simulink model "MT_FOC_control_autotuning"  (R2018a)
settings: Solver=ode4  StartTime=0.0  StopTime=3  FixedStep=1e-6  MaxStep=1e-4  RelTol=1e-3
undefined symbols (not defined in the file or in its folder): sigbuilder_block
libraries: powerlib x10, peTransforms x2, powerlib_meascontrol x1
settings Model: Creator=Admin  LastModifiedBy=Admin
settings DebuggingCC: MaxConsecutiveZCsMsg=none

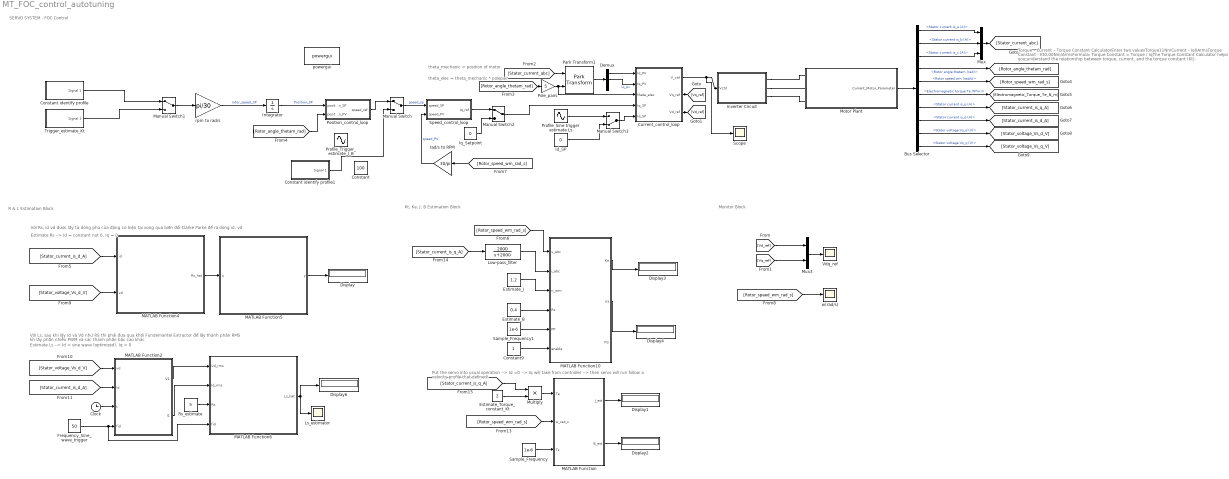
== system MT_FOC_control_autotuning ==
  note: Monitor Block
  note: Put the servo into usual operation --> Id =0 --> Iq will take from controller --> then servo will run follow a velocity profile that defined!
  note: Kt, Ke, J, B Estimation Block
  note: R & L Estimation Block
  note: Estimate Rs --> Id = constant not 0, Iq = 0
  note: SERVO SYSTEM - FOC Control
  note: Với Ls, sau khi lấy Id và Vd như RS thì phải đưa qua khối Fundemantel Extractor để lấy thành phần RMS kh lấy phần nhiễu PWM và các thành phần bậc cao khác
  note: Với Rs, id vd được lấy từ dòng pha của động cơ hiện tại xong qua biến đổi Clarke Parke để ra dòng id, vd
  note: Torque – Current – Torque Constant CalculatorEnter two valuesTorque11NmCurrent - Iq0ArmsTorque Constant - Kt0.00Nm/ArmsFormula: Torque Constant = Torque / IqThe Torque Constant Calculator helps you understand the relationship between torque, current, and the torque constant (Kt​).
  note: theta_mechanic = position of motor
  note: theta_elec = theta_mechanic * polepair
  note: Estimate Ls --> Id = sine wave (optimized), Iq = 0
  Bus Selector : BusSelector  OutputSignals=Stator current is_a (A),Stator current is_b (A),Stator current is_c (A),Rotor angle thetam (rad),Rotor speed wm (rad/s),Electromagnetic torque Te (N*m),Stator current is_q (A),Stator current is_d (A),Stator voltage Vs_d (V),Stator voltage Vs_q (V)
  Clock : Clock
  Constant : Constant  Value=100
  Constant identify profile : Subsystem  Tag=STV Subsys  LoadFcn=sigbuilder_block('load');  StartFcn=sigbuilder_block('start');  StopFcn=sigbuilder_block('stop');  ClipboardFcn=sigbuilder_block('clipboard');  mask(Sigbuilder block){tuvar=[0:10]}
      mask help: Simulink:masks:SigbuilderBlock_MD
      mask init:
      | if ~strcmp(get_param(bdroot(gcbh),'SimulationStatus'),'stopped') tuvar = sigbuilder_block('maskInit'); end
      settings: CopyFcn=sigbuilder_block('copy');  DeleteFcn=sigbuilder_block('delete');  ModelCloseFcn=sigbuilder_block('modelClose');  PreSaveFcn=sigbuilder_block('preSave');  PauseFcn=sigbuilder_block('pause');  ContinueFcn=sigbuilder_block('continue');  NameChangeFcn=sigbuilder_block('namechange');  OpenFcn=sigbuilder_block('open',[356.4 94.8 550.8 400.2 ]);  CloseFcn=sigbuilder_block('close');
      mask Display: plot(0, 0, 100, 100,[2, 2, 32, 32, 2], [68, 8, 8, 68, 68],[32, 2], [38, 38], [32, 19, 2],[53, 60, 44], [32, 17, 17, 2],[16, 16, 31, 31]);txt = getActiveGroup(gcbh);text(2, 100, txt,'verticalAlignment', 'top');
  Constant identify profile1 : Subsystem  Tag=STV Subsys  LoadFcn=sigbuilder_block('load');  StartFcn=sigbuilder_block('start');  StopFcn=sigbuilder_block('stop');  ClipboardFcn=sigbuilder_block('clipboard');  mask(Sigbuilder block){tuvar=[0:10]}
      mask help: Simulink:masks:SigbuilderBlock_MD
      mask init:
      | if ~strcmp(get_param(bdroot(gcbh),'SimulationStatus'),'stopped') tuvar = sigbuilder_block('maskInit'); end
      settings: CopyFcn=sigbuilder_block('copy');  DeleteFcn=sigbuilder_block('delete');  ModelCloseFcn=sigbuilder_block('modelClose');  PreSaveFcn=sigbuilder_block('preSave');  PauseFcn=sigbuilder_block('pause');  ContinueFcn=sigbuilder_block('continue');  NameChangeFcn=sigbuilder_block('namechange');  OpenFcn=sigbuilder_block('open',[356.4 94.8 550.8 400.2 ]);  CloseFcn=sigbuilder_block('close');
      mask Display: plot(0, 0, 100, 100,[2, 2, 32, 32, 2], [68, 8, 8, 68, 68],[32, 2], [38, 38], [32, 19, 2],[53, 60, 44], [32, 17, 17, 2],[16, 16, 31, 31]);txt = getActiveGroup(gcbh);text(2, 100, txt,'verticalAlignment', 'top');
  Constant9 : Constant
  Current_control_loop : Subsystem  mask{Kp=100, Ki=10}
  Demux : Demux  Outputs=3
  Display{,1..4,6} (6 alike) : Display
  Estimate_B : Constant  Value=0.4
  Estimate_J : Constant  Value=1.2
  "Estimate_Torque_constant_Kt " : Constant  Value=2  VectorParams1D=off  SampleTime=-1
  Frequency_Sine_wave_trigger : Constant  Value=50
  Id_SP : Constant  Value=0
  Integrator : Integrator
  Inverter Circuit : Subsystem  mask{Vdc=300, f_triangle=10000}
      mask prompts: Vdc "DC supply"; f_triangle "Freq carry signal"
  Iq_Setpoint : Constant  Value=0
  Low-pass_filter : TransferFcn  Numerator=[2000]  Denominator=[1 2000]
  Ls_estimator : Scope
  MATLAB Function : MATLAB Function  TreatAsAtomicUnit=on
  MATLAB Function10 : MATLAB Function  TreatAsAtomicUnit=on
  MATLAB Function2 : MATLAB Function  TreatAsAtomicUnit=on
  MATLAB Function4 : MATLAB Function  TreatAsAtomicUnit=on
  MATLAB Function5 : MATLAB Function  TreatAsAtomicUnit=on
  MATLAB Function6 : MATLAB Function  TreatAsAtomicUnit=on
  Manual Switch : ManualSwitch
  Manual Switch1 : ManualSwitch
  Manual Switch2 : ManualSwitch
  Manual Switch3 : ManualSwitch  CurrentSetting=0
  Motor Plant : Subsystem  mask{Load=0, Stator_Rs=2.4, L=0.00334, Torque_constant=0.2, pole_pairs=5, Intertia=0.000034, B=0}
      mask prompts: Load "Input load to Motor? (N.m)"; Stator_Rs "Stator phase resistance Rs (ohm)?"; L "Stator Armature inductance (H)?"; Torque_constant "Torque_constant? (N.m/A_peak)"; pole_pairs "Pole_pairs? (np)"; Intertia "Intertia (kg.m^2)"; B "Statis friction constant (N.m.s)"
  Multiply : Product
  Mux : Mux  Inputs=3
  Mux3 : Mux  Inputs=2
  Park Transform1 : peTransforms/Park Transform  AxisAlignment=Q-axis  PowerInvariant=off
  Pole_pairs : Gain  Gain=5
  Position_control_loop : Subsystem  mask{Kp=100, Ki=10, Feed_Fw_gain=1}
  Profile_Sine trigger estimate Ls : Sin  Amplitude=3  Frequency=100*pi  SampleTime=0
  Profile_Trigger_estimate_J_B : Sin  Amplitude=100  SampleTime=0
  Rs_estimate : Constant  Value=5
  Sample_Frequency : Constant  Value=1e-6
  Sample_Frequency1 : Constant  Value=1e-6
  Scope : Scope
  Speed_control_loop : Subsystem  mask{Kp=100, Ki=10}
  Trigger_estimate_Kt : Subsystem  Tag=STV Subsys  LoadFcn=sigbuilder_block('load');  StartFcn=sigbuilder_block('start');  StopFcn=sigbuilder_block('stop');  ClipboardFcn=sigbuilder_block('clipboard');  mask(Sigbuilder block){tuvar=[0:10]}
      mask help: Simulink:masks:SigbuilderBlock_MD
      mask init:
      | if ~strcmp(get_param(bdroot(gcbh),'SimulationStatus'),'stopped') tuvar = sigbuilder_block('maskInit'); end
      settings: CopyFcn=sigbuilder_block('copy');  DeleteFcn=sigbuilder_block('delete');  ModelCloseFcn=sigbuilder_block('modelClose');  PreSaveFcn=sigbuilder_block('preSave');  PauseFcn=sigbuilder_block('pause');  ContinueFcn=sigbuilder_block('continue');  NameChangeFcn=sigbuilder_block('namechange');  OpenFcn=sigbuilder_block('open',[356.4 94.8 550.8 400.2 ]);  CloseFcn=sigbuilder_block('close');
      mask Display: plot(0, 0, 100, 100,[2, 2, 32, 32, 2], [68, 8, 8, 68, 68],[32, 2], [38, 38], [32, 19, 2],[53, 60, 44], [32, 17, 17, 2],[16, 16, 31, 31]);txt = getActiveGroup(gcbh);text(2, 100, txt,'verticalAlignment', 'top');
  Vdq_ref : Scope
  powergui : powerlib/powergui  Priority=1  SimulationMode=Discrete  SampleTime=1e-6  frequency=60  Iterations=50  frequencyindice=0  Pbase=100e6  ErrMax=1e-4  UnitsV=kV  UnitsW=MW  buscounter=0  FunctionMessages=off  echomessages=off  EnableUseOfTLC=off  CurrentSourceSwitches=off  DisableSnubberDevices=off  DisableRonSwitches=off  DisableVfSwitches=off  DisplayEquations=off  SolverType=Tustin/Backward Euler (TBE)  Interpol=off  ExternalGateDelay=off  methode=off  Ts=100  x0status=blocks  SPID=on  SwTol=0  HookPort=off  RestoreLinks=warning  ResistiveCurrentMeasurement=off  Frange=[0:2:500]  Ylog=off  Xlog=on  ShowGrid=off  save=off  variable=ZData  structure=0  ZoomFFT=off  StartTime=0.0  cycles=1  DisplayStyle=1  fundamental=60  FreqAxis=off  MaxFrequency=1000  frequencyindicesteady=1  RmsSteady=1  display=off
  rad/s to RPM : Gain  Gain=30/pi
  rpm to rad/s : Gain  Gain=pi/30
  w(rad/s) : Scope
  wires:
  Bus Selector/1 -> Mux/1  "<Stator current is_a (A)>"
  Bus Selector/2 -> Mux/2  "<Stator current is_b (A)>"
  Bus Selector/3 -> Mux/3  "<Stator current is_c (A)>"
  Pole_pairs/1 -> Current_control_loop/3("theta_elec "), Park Transform1/2
  Park Transform1/1 -> Demux/1
  rpm to rad/s/1 -> Integrator/1  "rotor_speed_SP"
  Integrator/1 -> Position_control_loop/1(position_SP)  "Position_SP"
  Position_control_loop/1(speed_ref) -> Manual Switch/1
  Bus Selector/6 -> [Electromagnetic_Torque_Te_N_m]  "<Electromagnetic torque Te (N*m)>"
  Sample_Frequency/1 -> MATLAB Function/3(Ts)
  Constant identify profile/1(Signal 1) -> Manual Switch1/1
  Manual Switch1/1 -> rpm to rad/s/1
  Speed_control_loop/1(Iq_ref) -> Manual Switch2/1
  Iq_Setpoint/1 -> Manual Switch2/2
  MATLAB Function4/1(Rs_hat) -> MATLAB Function5/1(u)
  Id_SP/1 -> Manual Switch3/2
  Profile_Sine trigger estimate Ls/1 -> Manual Switch3/1
  MATLAB Function6/1(Ls_hat) -> Display6/1, Ls_estimator/1
  Clock/1 -> MATLAB Function2/3(t)
  Low-pass_filter/1 -> MATLAB Function10/2(i_abc)
  Trigger_estimate_Kt/1(Signal 1) -> Manual Switch1/2
  Sample_Frequency1/1 -> MATLAB Function10/5(PP)
  Constant9/1 -> MATLAB Function10/6(enable)
  Motor Plant/1(Current_Motor_Parameter) -> Bus Selector/1
  [Vd_ref] -> Mux3/1
  Mux3/1 -> Vdq_ref/1
  [Vq_ref] -> Mux3/2
  Current_control_loop/1(V_ctrl) -> Scope/1, Inverter Circuit/1(Vctrl)
  Current_control_loop/2(Vq_ref) -> [Vq_ref]
  Current_control_loop/3(Vd_ref) -> [Vd_ref]
  [Stator_current_abc] -> Park Transform1/1
  Mux/1 -> [Stator_current_abc]
  Bus Selector/4 -> [Rotor_angle_thetam_rad]  "<Rotor angle thetam (rad)>"
  [Rotor_angle_thetam_rad] -> Pole_pairs/1
  [Rotor_angle_thetam_rad] -> Position_control_loop/2(position_PV)
  [Rotor_speed_wm_rad_s] -> MATLAB Function10/1(v_abc)
  [Rotor_speed_wm_rad_s] -> rad/s to RPM/1
  Bus Selector/5 -> [Rotor_speed_wm_rad_s]  "<Rotor speed wm (rad/s)>"
  [Rotor_speed_wm_rad_s] -> w(rad/s)/1
  Bus Selector/10 -> [Stator_voltage_Vs_q_V]  "<Stator voltage Vs_q (V)>"
  Bus Selector/8 -> [Stator_current_is_d_A]  "<Stator current is_d (A)>"
  Bus Selector/9 -> [Stator_voltage_Vs_d_V]  "<Stator voltage Vs_d (V)>"
  Bus Selector/7 -> [Stator_current_is_q_A]  "<Stator current is_q (A)>"
  Demux/1 -> Current_control_loop/1(Id_PV)
  Demux/2 -> Current_control_loop/2(Iq_PV)  "iq_pv"
  Manual Switch3/1 -> Current_control_loop/5(Id_SP)
  Manual Switch2/1 -> Current_control_loop/4(Iq_SP)
  rad/s to RPM/1 -> Speed_control_loop/2(speed_PV)  "speed_PV"
  Manual Switch/1 -> Speed_control_loop/1(speed_SP)  "speed_sp"
  [Stator_current_is_d_A] -> MATLAB Function4/1(id)
  [Stator_voltage_Vs_d_V] -> MATLAB Function4/2(vd)
  MATLAB Function5/1(y) -> Display/1
  Frequency_Sine_wave_trigger/1 -> MATLAB Function6/4(fid), MATLAB Function2/4(fid)
  [Stator_voltage_Vs_d_V] -> MATLAB Function2/1(vd)
  [Stator_current_is_d_A] -> MATLAB Function2/2(id)
  MATLAB Function2/1(V1) -> MATLAB Function6/1(Vd_rms)
  MATLAB Function2/2(I1) -> MATLAB Function6/2(Id_rms)
  Rs_estimate/1 -> MATLAB Function6/3(Rs)
  [Rotor_speed_wm_rad_s] -> MATLAB Function/2(w_rad_s)
  MATLAB Function/1(J_est) -> Display1/1
  MATLAB Function/2(B_est) -> Display2/1
  [Stator_current_is_q_A] -> Low-pass_filter/1
  Multiply/1 -> MATLAB Function/1(Te)
  "Estimate_Torque_constant_Kt "/1 -> Multiply/2
  [Stator_current_is_q_A] -> Multiply/1
  MATLAB Function10/1(Ke) -> Display3/1
  MATLAB Function10/2(Kt) -> Display4/1
  Estimate_B/1 -> MATLAB Function10/4(Rs)
  Estimate_J/1 -> MATLAB Function10/3(n_rpm)
  Constant identify profile1/1(Signal 1) -> Manual Switch/2
  connections:
  Inverter Circuit/RConn1 -- Motor Plant/LConn1
  Inverter Circuit/RConn2 -- Motor Plant/LConn2
  Inverter Circuit/RConn3 -- Motor Plant/LConn3

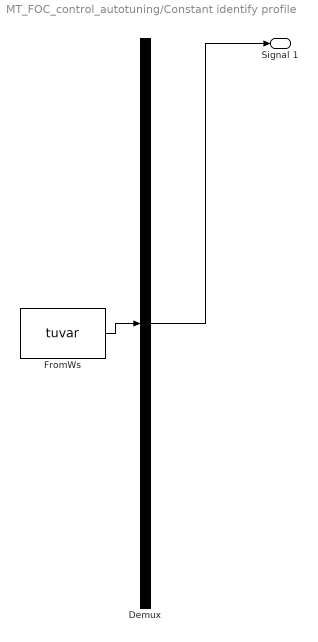
== system MT_FOC_control_autotuning/Constant identify profile ==
  Demux : Demux  Tag=STV Demux  Outputs=1
  FromWs : FromWorkspace  Tag=STV FromWs  VariableName=tuvar  SampleTime=0
      SigBuilderData=|
      | common.afterFinalStr = 'Extrapolate'
      | common.sampleTime = 0
      | dataSet.timeRange = [0 3]
      | dataSet.name = 'Group 1'
      | sbobj.Groups.Name = 'Group 1'
      | sbobj.Groups.Signals.Name = 'Signal 1'
      | sbobj.Groups.Signals.XData = [0 0.2 0.6 0.8 1.2 1.44 1.605 2.24 3]
      | sbobj.Groups.Signals.YData = [0.005 200 200 0 -0.5 99.5 99.5 0 0.005]
      | sbobj.Groups.TimeRange = [0 3]
  Signal 1 : Outport  Tag=STV Outport
  wires:
  Demux/1 -> Signal 1/1
  FromWs/1 -> Demux/1

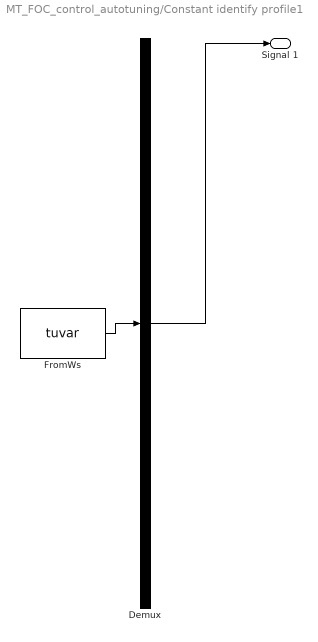
== system MT_FOC_control_autotuning/Constant identify profile1 ==
  Demux : Demux  Tag=STV Demux  Outputs=1
  FromWs : FromWorkspace  Tag=STV FromWs  VariableName=tuvar  SampleTime=0
      SigBuilderData=|
      | common.afterFinalStr = 'Extrapolate'
      | common.sampleTime = 0
      | dataSet.timeRange = [0 3]
      | dataSet.name = 'Group 1'
      | sbobj.Groups.Name = 'Group 1'
      | sbobj.Groups.Signals.Name = 'Signal 1'
      | sbobj.Groups.Signals.XData = [0 0.2 0.6 0.8 1.2 1.44 1.605 2.24 3]
      | sbobj.Groups.Signals.YData = [0.005 200 200 0 -0.5 99.5 99.5 0 0.005]
      | sbobj.Groups.TimeRange = [0 3]
  Signal 1 : Outport  Tag=STV Outport
  wires:
  Demux/1 -> Signal 1/1
  FromWs/1 -> Demux/1

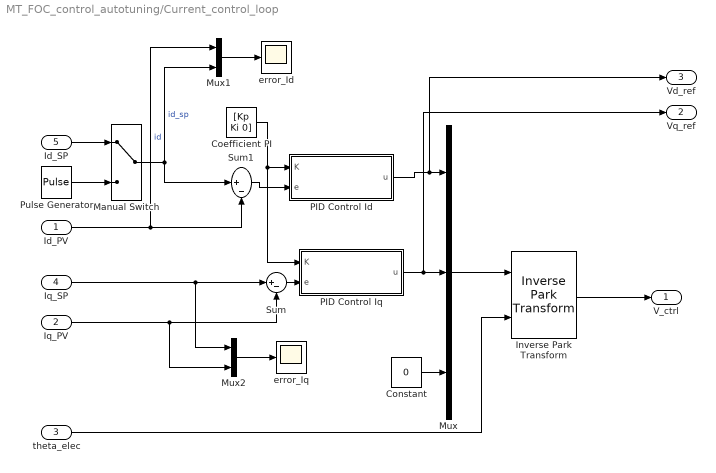
== system MT_FOC_control_autotuning/Current_control_loop ==
  Id_PV : Inport
  Iq_PV : Inport  Port=2
  "theta_elec " : Inport  Port=3
  Iq_SP : Inport  Port=4
  Id_SP : Inport  Port=5
  Coefficient PI : Constant  Value=[Kp Ki 0]
  Constant : Constant  Value=0
  Inverse Park Transform : peTransforms/Inverse Park Transform  AxisAlignment=Q-axis  PowerInvariant=off
  Manual Switch : ManualSwitch
  Mux : Mux  Inputs=3
  Mux1 : Mux  Inputs=2
  Mux2 : Mux  Inputs=2
  PID Control Id : Subsystem
  PID Control Iq : Subsystem
  Pulse Generator : DiscretePulseGenerator  PulseType=Time based  Period=0.01  PulseWidth=50
  Sum : Sum  Inputs=|+-
  Sum1 : Sum  Inputs=|+-
  error_Id : Scope
  error_Iq : Scope
  V_ctrl : Outport
  Vq_ref : Outport  Port=2
  Vd_ref : Outport  Port=3
  wires:
  Id_PV/1 -> Sum1/2, Mux1/1  "id"
  Sum1/1 -> PID Control Id/2(e)
  Inverse Park Transform/1 -> V_ctrl/1
  Iq_SP/1 -> Mux2/1, Sum/1
  Iq_PV/1 -> Mux2/2, Sum/2
  Sum/1 -> PID Control Iq/2(e)
  Coefficient PI/1 -> PID Control Iq/1(K), PID Control Id/1(K)
  PID Control Iq/1(u) -> Vq_ref/1, Mux/2
  Pulse Generator/1 -> Manual Switch/2
  Manual Switch/1 -> Sum1/1, Mux1/2  "id_sp"
  Mux1/1 -> error_Id/1
  Id_SP/1 -> Manual Switch/1
  Mux2/1 -> error_Iq/1
  Mux/1 -> Inverse Park Transform/1
  Constant/1 -> Mux/3
  "theta_elec "/1 -> Inverse Park Transform/2
  PID Control Id/1(u) -> Vd_ref/1, Mux/1

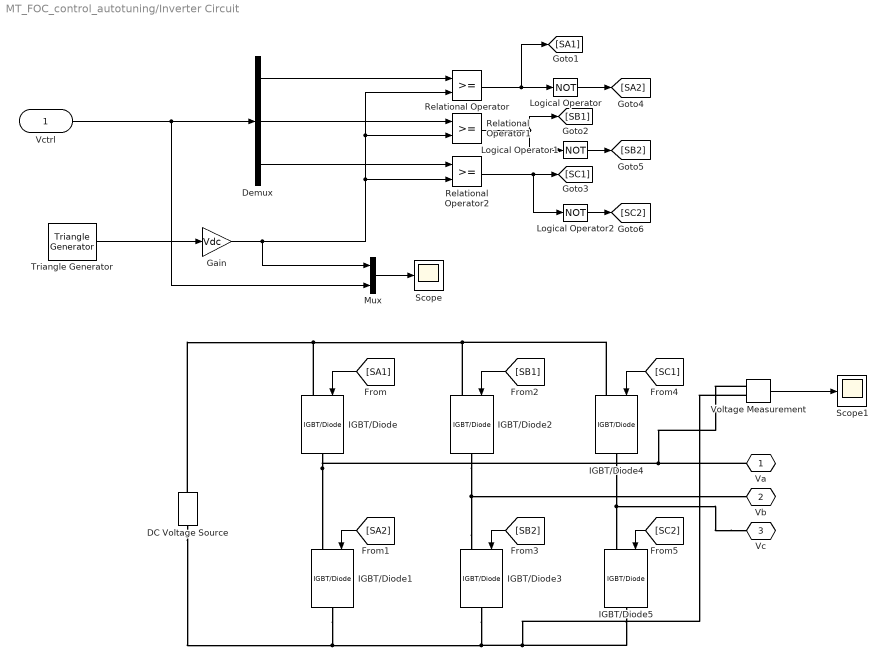
== system MT_FOC_control_autotuning/Inverter Circuit ==
  Vctrl : Inport
  DC Voltage Source : powerlib/Electrical Sources/DC Voltage Source  Amplitude=Vdc  Measurements=Voltage
  Demux : Demux  Outputs=3
  Gain : Gain  Gain=Vdc
  IGBT/Diode{,1..5} (6 alike) : powerlib/Power Electronics/IGBT//Diode  Ron=1e-3  Rs=1e5  Cs=inf  Measurements=off
  Logical Operator : Logic  Operator=NOT  AllPortsSameDT=off  OutDataTypeStr=boolean
  Logical Operator1 : Logic  Operator=NOT  AllPortsSameDT=off  OutDataTypeStr=boolean
  Logical Operator2 : Logic  Operator=NOT  AllPortsSameDT=off  OutDataTypeStr=boolean
  Mux : Mux  Inputs=2
  Relational Operator : RelationalOperator  OutDataTypeStr=boolean  RndMeth=Nearest
  Relational Operator1 : RelationalOperator  OutDataTypeStr=boolean  RndMeth=Nearest
  Relational Operator2 : RelationalOperator  OutDataTypeStr=boolean  RndMeth=Nearest
  Scope : Scope
  Scope1 : Scope
  Triangle Generator : powerlib_meascontrol/Pulse & Signal Generators/Triangle Generator  Freq=f_triangle  Phase=90  Ts=1e-6
  Voltage Measurement : powerlib/Measurements/Voltage Measurement  PhasorSimulation=off  OutputType=Complex  PSBequivalent=0
  Va : PMIOPort  Tag=PMCPort  Side=Right
  Vb : PMIOPort  Tag=PMCPort  Port=2  Side=Right
  Vc : PMIOPort  Tag=PMCPort  Port=3  Side=Right
  wires:
  Demux/1 -> Relational Operator/1
  Logical Operator2/1 -> [SC2]
  [SC1] -> IGBT/Diode4/1
  [SB1] -> IGBT/Diode2/1
  [SA1] -> IGBT/Diode/1
  [SB2] -> IGBT/Diode3/1
  Demux/2 -> Relational Operator1/1
  Relational Operator2/1 -> Logical Operator2/1, [SC1]
  Relational Operator/1 -> [SA1], Logical Operator/1
  Gain/1 -> Mux/1, Relational Operator2/2, Relational Operator1/2, Relational Operator/2
  Relational Operator1/1 -> Logical Operator1/1, [SB1]
  Demux/3 -> Relational Operator2/1
  [SA2] -> IGBT/Diode1/1
  Triangle Generator/1 -> Gain/1
  Logical Operator1/1 -> [SB2]
  Logical Operator/1 -> [SA2]
  Vctrl/1 -> Mux/2, Demux/1
  [SC2] -> IGBT/Diode5/1
  Mux/1 -> Scope/1
  Voltage Measurement/1 -> Scope1/1
  connections:
  IGBT/Diode3/LConn1 -- IGBT/Diode2/RConn1 -- Vb/RConn1
  IGBT/Diode/LConn1 -- DC Voltage Source/RConn1 -- IGBT/Diode2/LConn1 -- IGBT/Diode4/LConn1
  IGBT/Diode5/RConn1 -- Voltage Measurement/LConn2 -- IGBT/Diode3/RConn1 -- DC Voltage Source/LConn1 -- IGBT/Diode1/RConn1
  Vc/RConn1 -- IGBT/Diode4/RConn1 -- IGBT/Diode5/LConn1
  Va/RConn1 -- Voltage Measurement/LConn1 -- IGBT/Diode/RConn1 -- IGBT/Diode1/LConn1

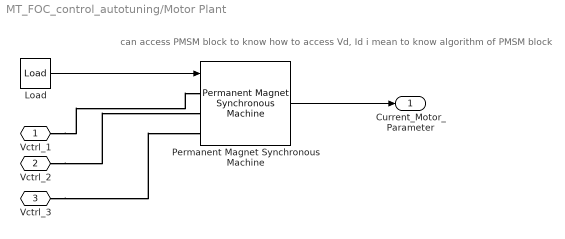
== system MT_FOC_control_autotuning/Motor Plant ==
  note: can access PMSM block to know how to access Vd, Id i mean to know algorithm of PMSM block
  Load : Constant  Value=Load
  Permanent Magnet Synchronous Machine : powerlib/Machines/Permanent Magnet Synchronous Machine  NbPhases=3  FluxDistribution=Sinusoidal  RotorType=Round  MechanicalLoad=Torque Tm  PresetModel=No  ShowDetailedParameters=on  MeasurementBus=off  Resistance=Stator_Rs  Inductance=8.5e-3  dqInductances=[8.5e-3,8.5e-3]  La=L  MachineConstant=Torque Constant (N.m / A_peak)  Flux=0.026667  VoltageCst=24.184  TorqueCst=Torque_constant  Flat=120  Mechanical=[Intertia B pole_pairs 0]  PolePairs=2  InitialConditions=[0,0, 0,0]  InitialConditions5ph=[0 0 0 0 0 0]  TsPowergui=0  TsBlock=-1  RefAngle=90 degrees behind phase A axis (modified Park)
      settings: SourceProductName=Simscape Power Systems
  Vctrl_1 : PMIOPort  Side=Left
  Vctrl_2 : PMIOPort  Port=2  Side=Left
  Vctrl_3 : PMIOPort  Port=3  Side=Left
  Current_Motor_Parameter : Outport
  wires:
  Load/1 -> Permanent Magnet Synchronous Machine/1
  Permanent Magnet Synchronous Machine/1 -> Current_Motor_Parameter/1
  connections:
  Vctrl_2/RConn1 -- Permanent Magnet Synchronous Machine/LConn2
  Vctrl_1/RConn1 -- Permanent Magnet Synchronous Machine/LConn1
  Vctrl_3/RConn1 -- Permanent Magnet Synchronous Machine/LConn3

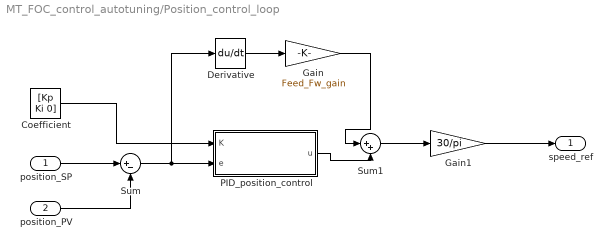
== system MT_FOC_control_autotuning/Position_control_loop ==
  position_SP : Inport
  position_PV : Inport  Port=2
  Coefficient : Constant  Value=[Kp Ki 0]
  Derivative : Derivative
  Gain : Gain  Gain=Feed_Fw_gain
  Gain1 : Gain  Gain=30/pi
  PID_position_control : Subsystem
  Sum : Sum  Inputs=|+-
  Sum1 : Sum  Inputs=|++
  speed_ref : Outport
  wires:
  Coefficient/1 -> PID_position_control/1(K)
  position_SP/1 -> Sum/1
  position_PV/1 -> Sum/2
  Sum/1 -> Derivative/1, PID_position_control/2(e)
  Derivative/1 -> Gain/1
  Gain/1 -> Sum1/1
  PID_position_control/1(u) -> Sum1/2
  Sum1/1 -> Gain1/1
  Gain1/1 -> speed_ref/1

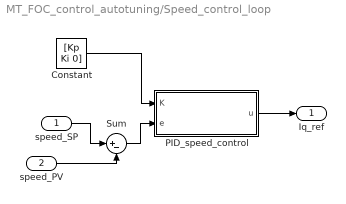
== system MT_FOC_control_autotuning/Speed_control_loop ==
  speed_SP : Inport
  speed_PV : Inport  Port=2
  Constant : Constant  Value=[Kp Ki 0]
  PID_speed_control : Subsystem
  Sum : Sum  Inputs=|+-
  Iq_ref : Outport
  wires:
  Constant/1 -> PID_speed_control/1(K)
  PID_speed_control/1(u) -> Iq_ref/1
  speed_SP/1 -> Sum/1
  speed_PV/1 -> Sum/2
  Sum/1 -> PID_speed_control/2(e)

== system MT_FOC_control_autotuning/Trigger_estimate_Kt ==
  Demux : Demux  Tag=STV Demux  Outputs=1
  FromWs : FromWorkspace  Tag=STV FromWs  VariableName=tuvar  SampleTime=0
      SigBuilderData=|
      | common.afterFinalStr = 'Extrapolate'
      | common.sampleTime = 0
      | dataSet.timeRange = [0 3]
      | dataSet.name = 'Group 1'
      | sbobj.Groups.Name = 'Group 1'
      | sbobj.Groups.Signals.Name = 'Signal 1'
      | sbobj.Groups.Signals.XData = [0 0.2 0.6 0.8 1.2 1.44 1.605 2.24 3]
      | sbobj.Groups.Signals.YData = [0.005 78 230 302 434 522 596 794 795]
      | sbobj.Groups.TimeRange = [0 3]
  Signal 1 : Outport  Tag=STV Outport
  wires:
  Demux/1 -> Signal 1/1
  FromWs/1 -> Demux/1

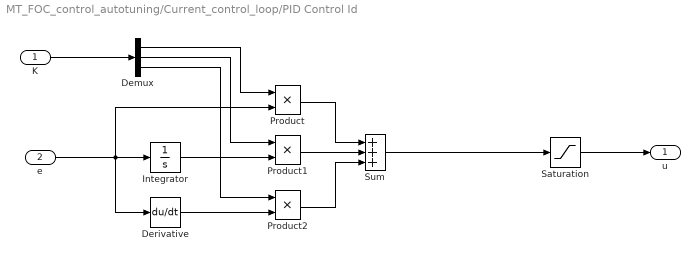
== system MT_FOC_control_autotuning/Current_control_loop/PID Control Id ==
  K : Inport
  e : Inport  Port=2
  Demux : Demux  Outputs=3
  Derivative : Derivative
  Integrator : Integrator
  Product : Product  SaturateOnIntegerOverflow=on  OutDataTypeStr=Inherit: Same as first input
  Product1 : Product  SaturateOnIntegerOverflow=on  OutDataTypeStr=Inherit: Same as first input
  Product2 : Product  SaturateOnIntegerOverflow=on  OutDataTypeStr=Inherit: Same as first input
  Saturation : Saturate  UpperLimit=200  LowerLimit=-200
  Sum : Sum  Inputs=+++  SaturateOnIntegerOverflow=on  InputSameDT=on  OutDataTypeStr=Inherit: Same as first input
  u : Outport
  wires:
  Demux/2 -> Product1/1
  Demux/1 -> Product/1
  Demux/3 -> Product2/1
  e/1 -> Product/2, Integrator/1, Derivative/1
  Product2/1 -> Sum/3
  Integrator/1 -> Product1/2
  Derivative/1 -> Product2/2
  Product/1 -> Sum/1
  K/1 -> Demux/1
  Product1/1 -> Sum/2
  Sum/1 -> Saturation/1
  Saturation/1 -> u/1

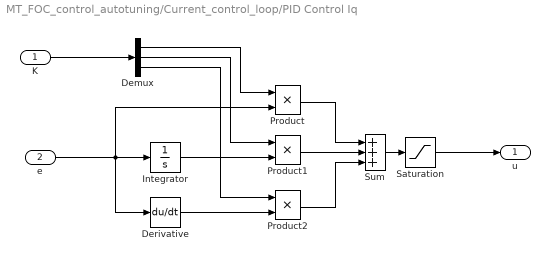
== system MT_FOC_control_autotuning/Current_control_loop/PID Control Iq ==
  K : Inport
  e : Inport  Port=2
  Demux : Demux  Outputs=3
  Derivative : Derivative
  Integrator : Integrator
  Product : Product  SaturateOnIntegerOverflow=on  OutDataTypeStr=Inherit: Same as first input
  Product1 : Product  SaturateOnIntegerOverflow=on  OutDataTypeStr=Inherit: Same as first input
  Product2 : Product  SaturateOnIntegerOverflow=on  OutDataTypeStr=Inherit: Same as first input
  Saturation : Saturate  UpperLimit=200  LowerLimit=-200
  Sum : Sum  Inputs=+++  SaturateOnIntegerOverflow=on  InputSameDT=on  OutDataTypeStr=Inherit: Same as first input
  u : Outport
  wires:
  Demux/2 -> Product1/1
  Demux/1 -> Product/1
  Demux/3 -> Product2/1
  e/1 -> Product/2, Integrator/1, Derivative/1
  Product2/1 -> Sum/3
  Integrator/1 -> Product1/2
  Derivative/1 -> Product2/2
  Product/1 -> Sum/1
  K/1 -> Demux/1
  Product1/1 -> Sum/2
  Sum/1 -> Saturation/1
  Saturation/1 -> u/1

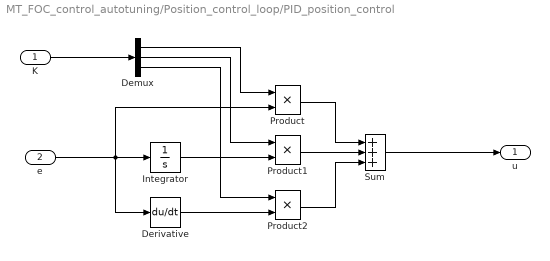
== system MT_FOC_control_autotuning/Position_control_loop/PID_position_control ==
  K : Inport
  e : Inport  Port=2
  Demux : Demux  Outputs=3
  Derivative : Derivative
  Integrator : Integrator
  Product : Product  SaturateOnIntegerOverflow=on  OutDataTypeStr=Inherit: Same as first input
  Product1 : Product  SaturateOnIntegerOverflow=on  OutDataTypeStr=Inherit: Same as first input
  Product2 : Product  SaturateOnIntegerOverflow=on  OutDataTypeStr=Inherit: Same as first input
  Sum : Sum  Inputs=+++  SaturateOnIntegerOverflow=on  InputSameDT=on  OutDataTypeStr=Inherit: Same as first input
  u : Outport
  wires:
  Demux/2 -> Product1/1
  Demux/1 -> Product/1
  Demux/3 -> Product2/1
  e/1 -> Product/2, Integrator/1, Derivative/1
  Product2/1 -> Sum/3
  Integrator/1 -> Product1/2
  Derivative/1 -> Product2/2
  Product/1 -> Sum/1
  K/1 -> Demux/1
  Product1/1 -> Sum/2
  Sum/1 -> u/1

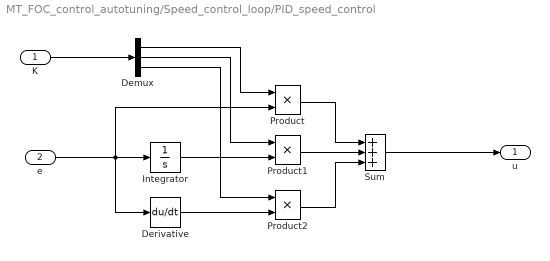
== system MT_FOC_control_autotuning/Speed_control_loop/PID_speed_control ==
  K : Inport
  e : Inport  Port=2
  Demux : Demux  Outputs=3
  Derivative : Derivative
  Integrator : Integrator
  Product : Product  SaturateOnIntegerOverflow=on  OutDataTypeStr=Inherit: Same as first input
  Product1 : Product  SaturateOnIntegerOverflow=on  OutDataTypeStr=Inherit: Same as first input
  Product2 : Product  SaturateOnIntegerOverflow=on  OutDataTypeStr=Inherit: Same as first input
  Sum : Sum  Inputs=+++  SaturateOnIntegerOverflow=on  InputSameDT=on  OutDataTypeStr=Inherit: Same as first input
  u : Outport
  wires:
  Demux/2 -> Product1/1
  Demux/1 -> Product/1
  Demux/3 -> Product2/1
  e/1 -> Product/2, Integrator/1, Derivative/1
  Product2/1 -> Sum/3
  Integrator/1 -> Product1/2
  Derivative/1 -> Product2/2
  Product/1 -> Sum/1
  K/1 -> Demux/1
  Product1/1 -> Sum/2
  Sum/1 -> u/1

== matlab function MT_FOC_control_autotuning/MATLAB Function ==
  data: Te input; J_est output; w_rad_s input; Ts input; B_est output
function [J_est, B_est] = Mechanical_Estimator(Te, w_rad_s, Ts)
    % Khai báo biến nhớ (Persistent variables) để lưu trạng thái giữa các bước
    persistent P theta w_prev
    
    % Khởi tạo lần đầu
    if isempty(P)
        P = 1000 * eye(2); % Ma trận hiệp phương sai ban đầu (lớn)
        theta = [0; 0];    % Vector tham số cần tìm [J; B]
        w_prev = 0;
    end
    
    % 1. Tính gia tốc (alpha) bằng đạo hàm số
    alpha = (w_rad_s - w_prev) / Ts;
    w_prev = w_rad_s;
    
    % Bỏ qua nếu gia tốc quá nhỏ (tránh chia cho 0 hoặc nhiễu)
    if abs(alpha) > 0.1 || abs(w_rad_s) > 0.1
        
        % 2. Xây dựng vector hồi quy (Regressor vector)
        % Phương trình: Te = J * alpha + B * w
        phi = [alpha; w_rad_s]; 
        
        % 3. Thuật toán RLS (Recursive Least Squares)
        % Tính sai số dự đoán
        e = Te - phi' * theta;
        
        % Tính Gain K
        K = P * phi / (1 + phi' * P * phi);
        
        % Cập nhật tham số theta [J; B]
        theta = theta + K * e;
        
        % Cập nhật ma trận P (Forgeting factor lambda = 0.999 cho mượt)
        lambda = 0.999;
        P = (P - K * phi' * P) / lambda;
    end
    
    % 4. Xuất kết quả
    J_est = theta(1);
    B_est = theta(2);
end

== matlab function MT_FOC_control_autotuning/MATLAB Function2 ==
  settings: updateMethod=DISCRETE
  data: vd input; V1 output; id input; t input; fid input; I1 output
function [V1, I1] = FundamentalExtractor(vd, id, t, fid)
% vd, id : tín hiệu PWM
% t      : thời gian
% fid    : tần số kích thích

w = 2*pi*fid;

persistent vsin vcos isin icos

if isempty(vsin)
    vsin = 0; vcos = 0;
    isin = 0; icos = 0;
end

vsin = vsin + vd * sin(w*t);
vcos = vcos + vd * cos(w*t);

isin = isin + id * sin(w*t);
icos = icos + id * cos(w*t);

V1 = 2*sqrt(vsin^2 + vcos^2);
I1 = 2*sqrt(isin^2 + icos^2);

== matlab function MT_FOC_control_autotuning/MATLAB Function4 ==
  settings: updateMethod=DISCRETE
  data: id input; vd input; Rs_hat output
function Rs_hat = estimate_Rs(id, vd)
% id, vd: vector tín hiệu đã đo trong trạng thái xác lập
% giả sử iq = 0, wm = 0

Rs_hat = mean(vd) / mean(id);
end

== matlab function MT_FOC_control_autotuning/MATLAB Function5 ==
  settings: updateMethod=DISCRETE
  data: u input; y output
function y = Mean_Filter(u)
% u : tín hiệu đầu vào (có ripple)
% y : giá trị trung bình (DC component)

persistent buf idx N

if isempty(buf)
    N = 1000;            % số mẫu trung bình (chỉnh được)
    buf = zeros(1, N);
    idx = 1;
end

buf(idx) = u;
idx = idx + 1;
if idx > N
    idx = 1;
end

y = mean(buf);

== matlab function MT_FOC_control_autotuning/MATLAB Function6 ==
  settings: updateMethod=DISCRETE
  data: Vd_rms input; Id_rms input; Ls_hat output; Rs input; fid input
function Ls_hat = Estimate_Ls_RMS(Vd_rms, Id_rms, Rs, fid)

w = 2*pi*fid;

Z = Vd_rms / Id_rms;

delta = Z^2 - Rs^2;

if delta > 0
    Ls_hat = sqrt(delta) / w;
else
    Ls_hat = 0;
end

== matlab function MT_FOC_control_autotuning/MATLAB Function10 ==
  settings: updateMethod=DISCRETE
  data: v_abc input; i_abc input; n_rpm input; Rs input; PP input; Ke output; enable input; Kt output; Psi output
function [Ke, Kt, Psi] = fcn(v_abc, i_abc, n_rpm, Rs, PP, enable)
    persistent v_sq_sum i_sq_sum speed_sum sample_count
    
    if isempty(v_sq_sum)
        v_sq_sum = 0; 
        i_sq_sum = 0; 
        speed_sum = 0; 
        sample_count = 0;
    end

    Ke = 0; Kt = 0; Psi = 0;

    if enable > 0
        v_ms_instant = (v_abc(1)^2 + v_abc(2)^2 + v_abc(3)^2) / 3;
        i_ms_instant = (i_abc(1)^2 + i_abc(2)^2 + i_abc(3)^2) / 3;
        
        v_sq_sum = v_sq_sum + v_ms_instant;
        i_sq_sum = i_sq_sum + i_ms_instant;
        speed_sum = speed_sum + abs(n_rpm);
        sample_count = sample_count + 1;
    else
        if sample_count > 0
            V_rms = sqrt(v_sq_sum / sample_count);
            I_rms = sqrt(i_sq_sum / sample_count);
            Avg_RPM = speed_sum / sample_count;
            
            V_bemf_rms_sq = V_rms^2 - (I_rms * Rs)^2;
            
            if V_bemf_rms_sq > (V_rms^2 * 0.05)
                V_bemf_rms = sqrt(V_bemf_rms_sq);
            else
                V_bemf_rms = V_rms;
            end
            
            omega_e = (2 * pi * Avg_RPM * PP) / 60;
            
            if omega_e > 0.1
                Psi_val = (V_bemf_rms * sqrt(2)) / omega_e;
                Psi = Psi_val;
                Ke = Psi_val;
                Kt = 1.5 * PP * Psi_val;
            end
            
            v_sq_sum = 0; 
            i_sq_sum = 0; 
            speed_sum = 0; 
            sample_count = 0;
        end
    end
end
